simulink model "v2test"  (R2020b)
settings: Solver=VariableStepAuto  StartTime=0.0  StopTime=1  RelTol=1e-3
undefined symbols (not defined in the file or in its folder): spacar_lib, SPASIM
settings Model: Creator=Rick  LastModifiedBy=Rick

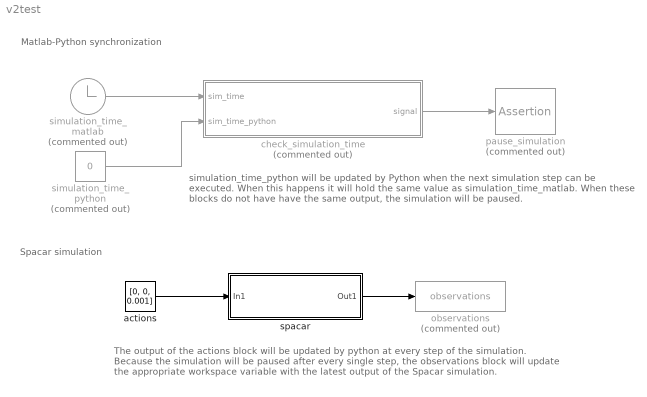
== system v2test ==
  note: The output of the actions block will be updated by python at every step of the simulation. Because the simulation will be paused after every single step, the observations block will update the appropriate workspace variable with the latest output of the Spacar simulation.
  note: simulation_time_python will be updated by Python when the next simulation step can be executed. When this happens it will hold the same value as simulation_time_matlab. When these blocks do not have have the same output, the simulation will be paused.
  note: Spacar simulation
  note: Matlab-Python synchronization
  actions : Constant  Value=[0, 0, 0.001]
  check_simulation_time : MATLAB Function  Commented=on  TreatAsAtomicUnit=on
  observations : ToWorkspace  Commented=on  VariableName=observations  SampleTime=-1
      settings: MaxDataPoints=1
  pause_simulation : Assertion  Commented=on  AssertionFailFcn=set_param(bdroot, 'SimulationCommand', 'pause')  StopWhenAssertionFail=off
  simulation_time_matlab : Clock  Commented=on
  simulation_time_python : Constant  Commented=on  Value=0
  spacar : Subsystem  AncestorBlock=spacar_lib/SPASIM  mask{filename='bicycle', use_spadraw=off, output_sbd=off}
      mask prompts: filename "SPACAR data filename"; use_spadraw "Visualize with spadraw"; output_sbd "Write SBD file"
      mask init:
      | if size(who('filenm'))>0; dfilenm=filenm; else; dfilenm=''; end
      mask Display: disp(filename);
  wires:
  spacar/1(Out1) -> observations/1
  actions/1 -> spacar/1(In1)
  simulation_time_matlab/1 -> check_simulation_time/1(sim_time)
  simulation_time_python/1 -> check_simulation_time/2(sim_time_python)
  check_simulation_time/1(signal) -> pause_simulation/1

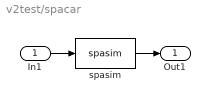
== system v2test/spacar ==
  In1 : Inport
  spasim : S-Function  FunctionName=spasim  Parameters=filename,use_spadraw,output_sbd  SFunctionDeploymentMode=off  EnableBusSupport=off
  Out1 : Outport  InitialOutput=0  VectorParamsAs1DForOutWhenUnconnected=off
  wires:
  spasim/1 -> Out1/1
  In1/1 -> spasim/1

== matlab function v2test/check_simulation_time ==
  data: sim_time input; sim_time_python input; signal output
function signal = assert_input(sim_time, sim_time_python)
    if sim_time > sim_time_python
        signal = 0; % pause sim until python let's it continue
    else if sim_time == sim_time_python
        signal = 1; % good to go
    else
        signal = 0;
        disp("Warning: Matlab' simulation is lagging behind Python.")
    end
end
